simulink model "ktest"  (Simulink 7.0)
settings: Solver=ode45  StartTime=0.0  StopTime=100000.0  RelTol=1e-3
undefined symbols (not defined in the file or in its folder): bit
libraries: c6713dsklib x3
settings Model: Creator=hp  LastModifiedBy=hp
settings OptimizationCC: OptimizeModelRefInitCode=on
settings RTWCC: SystemTargetFile=ccslink_ert.tlc  GenCodeOnly=on  GenerateMakefile=off  TemplateMakefile=ccslink_ert.tmf  Description=Link for CCS (ERT) code generation for TMS320(TM) DSP platforms  ProcessScript=ccslink_ert_make_rtw_hook
settings CodeAppCC: IgnoreCustomStorageClasses=off
settings ERTTgtLinkCCS: TargetFcnLib=ansi_tfl_table_tmw.mat  GenFloatMathFcnCalls=ANSI_C  UtilityFuncGeneration=Auto  GenerateFullHeader=on  GenerateSampleERTMain=off  GenerateTestInterfaces=off  IsPILTarget=off  ModelReferenceCompliant=on  CompOptLevelCompliant=off  IncludeMdlTerminateFcn=on  CombineOutputUpdateFcns=on  SuppressErrorStatus=off  IncludeFileDelimiter=Auto  ERTCustomFileBanners=on  SupportAbsoluteTime=on  LogVarNameModifier=rt_  MatFileLogging=off  MultiInstanceERTCode=off  SupportNonFinite=on  SupportComplex=on  PurelyIntegerCode=off  SupportContinuousTime=off  SupportNonInlinedSFcns=off  EnableShiftOperators=on  ParenthesesLevel=Nominal  PortableWordSizes=off  ModelStepFunctionPrototypeControlCompliant=off  GenerateErtSFunction=off  GenerateASAP2=off  ExtMode=off  ExtModeTransport=0  ExtModeStaticAlloc=off  ExtModeStaticAllocSize=1000000  ExtModeTesting=off  ExtModeMexFile=noextcomm  ExtModeIntrfLevel=Level1  InlinedParameterPlacement=NonHierarchical  TargetOS=BareBoardExample  MultiInstanceErrorCode=Error  RateGroupingCode=on  RootIOFormat=Individual arguments  RTWCAPISignals=off  RTWCAPIParams=off  RTWCAPIStates=off  ERTSrcFileBannerTemplate=ert_code_template.cgt  ERTHdrFileBannerTemplate=ert_code_template.cgt  ERTDataSrcFileTemplate=ert_code_template.cgt  ERTDataHdrFileTemplate=ert_code_template.cgt  ERTCustomFileTemplate=example_file_process.tlc  ModuleNamingRule=Unspecified  SignalDisplayLevel=10  ParamTuneLevel=10  GlobalDataDefinition=Auto  DataDefinitionFile=global.c  GlobalDataReference=Auto  DataReferenceFile=global.h  GRTInterface=off  PreserveExpressionOrder=off  PreserveIfCondition=off  EnableUserReplacementTypes=off  MemSecPackage=--- None ---  MemSecDataConstants=Default  MemSecDataIO=Default  MemSecDataInternal=Default  MemSecDataParameters=Default  MemSecFuncInitTerm=Default  MemSecFuncExecute=Default  exportIDEObj=on  ideObjName=CCS_Obj  oldideObjName=CCS_Obj  ProfileGenCode=off  ProfileNumSamples=100  InlineDSPBlks=on  projectOptions=Custom  debugCompilerOptions="-g -d\"_DEBUG\""  releaseCompilerOptions=-o2  getCompilerOptions=off  getLinkerOptions=off  systemStackSize=512  buildAction=Build_and_execute  overrunNotificationMethod=None  overrunNotificationFcn=myfunction  oldoverrunNotificationFcn=myfunction  configurePIL=off  configPILBlockAction=Create_PIL_block_build_and_download

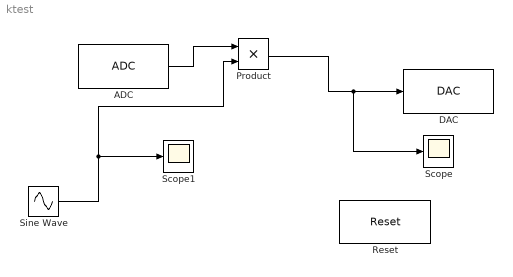
== system ktest ==
  ADC : c6713dsklib/ADC  ADCsource=Line In  MicGain=off  Stereo=on  SampleRate=8 kHz  CodecDataFormat=16-bit  OutputDataType=Integer  Scaling=Normalize  SourceGain=0.0  FrameSize=64  inheritSampleTime=off
  DAC : c6713dsklib/DAC  CodecDataFormat=16-bit  SampleRate=8 kHz  Scaling=Normalize  DacAtten=0.0  OverflowMode=Wrap
  Product : Product  OutDataType=sfix(16)  OutScaling=2^0  RndMeth=Zero
  Reset : c6713dsklib/Reset  SystemSampleTime=-1
  Scope : Scope
  Scope1 : Scope
  Sine Wave : Sin  Frequency=8000  SampleTime=0
  wires:
  ADC/1 -> Product/1
  Sine Wave/1 -> Product/2, Scope1/1
  Product/1 -> DAC/1, Scope/1
